simulink model "sus"  (Simulink 6.5)
settings: Solver=ode45  StartTime=0.0  StopTime=16  RelTol=1e-3
libraries: cdsFilt x266, cdsBitwise x92, cdsEpicsOut x84, cdsEpicsBinIn x56, cdsEpicsIn x20, cdsFiltCtrl x18, cdsMatrix x11, cdsSwitch x7, cdsWD x7, cdsFunctionCall x5, cdsRio1 x4, dac x3
(part 4 of 20)

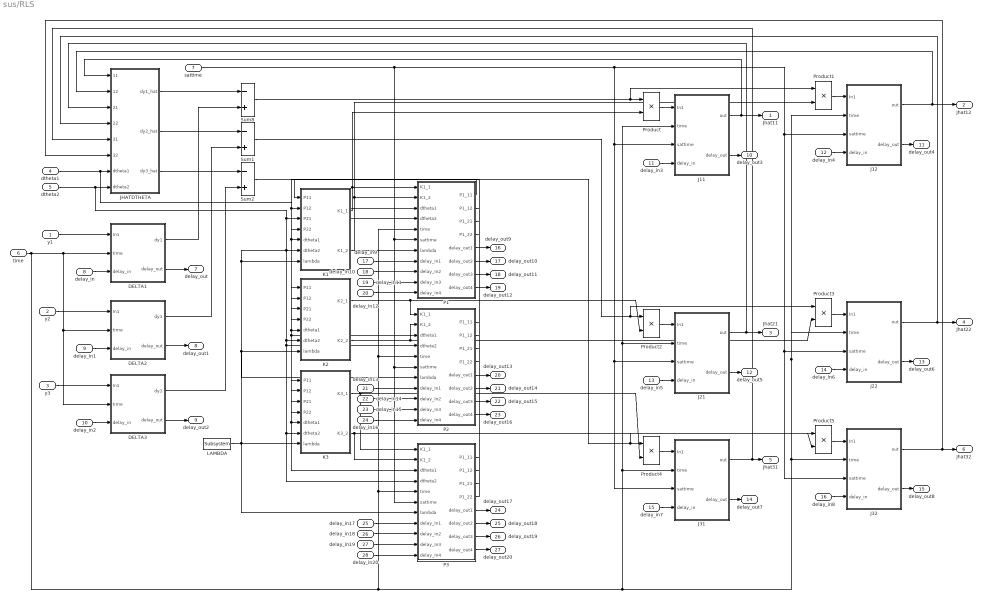
== system sus/RLS ==
  y1 : Inport
  y2 : Inport  Port=2
  y3 : Inport  Port=3
  dtheta1 : Inport  Port=4
  dtheta2 : Inport  Port=5
  time : Inport  Port=6
  sattime : Inport  Port=7
  delay_in : Inport  Port=8
  delay_in1 : Inport  Port=9
  delay_in2 : Inport  Port=10
  delay_in3 : Inport  Port=11
  delay_in4 : Inport  Port=12
  delay_in5 : Inport  Port=13
  delay_in6 : Inport  Port=14
  delay_in7 : Inport  Port=15
  delay_in8 : Inport  Port=16
  delay_in9 : Inport  Port=17
  delay_in10 : Inport  Port=18
  delay_in11 : Inport  Port=19
  delay_in12 : Inport  Port=20
  delay_in13 : Inport  Port=21
  delay_in14 : Inport  Port=22
  delay_in15 : Inport  Port=23
  delay_in16 : Inport  Port=24
  delay_in17 : Inport  Port=25
  delay_in18 : Inport  Port=26
  delay_in19 : Inport  Port=27
  delay_in20 : Inport  Port=28
  DELTA1 : Subsystem
  DELTA2 : Subsystem
  DELTA3 : Subsystem
  J11 : Subsystem
  J12 : Subsystem
  J21 : Subsystem
  J22 : Subsystem
  J31 : Subsystem
  J32 : Subsystem
  JHATDTHETA : Subsystem
  K1 : Subsystem
  K2 : Subsystem
  K3 : Subsystem
  LAMBDA : cdsEpicsIn/Subsystem  Tag=cdsEpicsIn  Description=|  SystemSampleTime=-1
      | Purpose:                                                                              
      | Create an EPICS input channel connection to the FE realtime controls.                 
      |                                                                                       
      | Operation:                                                                            
      | Outputs value from an EPICS ai record. Value is floating point with a precision of 3..
      |                                                                                       
      | Usage:                                                                                
      | Name the part with the desired EPICS channel name.
      settings: AttributesFormatString=%<Tag>
  P1 : Subsystem
  P2 : Subsystem
  P3 : Subsystem
  Product{,1..5} (6 alike) : Product  RndMeth=Zero
  Sum1 : Sum  Inputs=-+
  Sum2 : Sum  Inputs=-+
  Sum8 : Sum  Inputs=-+
  Jhat11 : Outport
  Jhat12 : Outport  Port=2
  Jhat21 : Outport  Port=3
  Jhat22 : Outport  Port=4
  Jhat31 : Outport  Port=5
  Jhat32 : Outport  Port=6
  delay_out : Outport  Port=7
  delay_out1 : Outport  Port=8
  delay_out2 : Outport  Port=9
  delay_out3 : Outport  Port=10
  delay_out4 : Outport  Port=11
  delay_out5 : Outport  Port=12
  delay_out6 : Outport  Port=13
  delay_out7 : Outport  Port=14
  delay_out8 : Outport  Port=15
  delay_out9 : Outport  Port=16
  delay_out10 : Outport  Port=17
  delay_out11 : Outport  Port=18
  delay_out12 : Outport  Port=19
  delay_out13 : Outport  Port=20
  delay_out14 : Outport  Port=21
  delay_out15 : Outport  Port=22
  delay_out16 : Outport  Port=23
  delay_out17 : Outport  Port=24
  delay_out18 : Outport  Port=25
  delay_out19 : Outport  Port=26
  delay_out20 : Outport  Port=27
  wires:
  time/1 -> DELTA1/2(time), DELTA2/2(time), DELTA3/2(time), J11/2(time), J21/2(time), J31/2(time), J12/2(time), J22/2(time), J32/2(time), P1/5(time), P2/5(time), P3/5(time)
  y1/1 -> DELTA1/1(In1)
  delay_in/1 -> DELTA1/3(delay_in)
  DELTA1/2(delay_out) -> delay_out/1
  y2/1 -> DELTA2/1(In1)
  delay_in1/1 -> DELTA2/3(delay_in)
  DELTA2/2(delay_out) -> delay_out1/1
  y3/1 -> DELTA3/1(In1)
  delay_in2/1 -> DELTA3/3(delay_in)
  DELTA3/2(delay_out) -> delay_out2/1
  dtheta1/1 -> JHATDTHETA/7(dtheta1), K1/5(dtheta1), K2/5(dtheta1), K3/5(dtheta1), P3/3(dtheta1), P2/3(dtheta1), P1/3(dtheta1)
  dtheta2/1 -> JHATDTHETA/8(dtheta2), K1/6(dtheta2), K2/6(dtheta2), K3/6(dtheta2), P3/4(dtheta2), P2/4(dtheta2), P1/4(dtheta2)
  JHATDTHETA/1(dy1_hat) -> Sum8/1
  DELTA1/1(dy1) -> Sum8/2
  JHATDTHETA/2(dy2_hat) -> Sum1/1
  DELTA2/1(dy1) -> Sum1/2
  JHATDTHETA/3(dy3_hat) -> Sum2/1
  DELTA3/1(dy1) -> Sum2/2
  delay_in3/1 -> J11/4(delay_in)
  J11/2(delay_out) -> delay_out3/1
  Product/1 -> J11/1(In1)
  delay_in4/1 -> J12/4(delay_in)
  J12/2(delay_out) -> delay_out4/1
  Product1/1 -> J12/1(In1)
  delay_in5/1 -> J21/4(delay_in)
  J21/2(delay_out) -> delay_out5/1
  Product2/1 -> J21/1(In1)
  delay_in6/1 -> J22/4(delay_in)
  J22/2(delay_out) -> delay_out6/1
  Product3/1 -> J22/1(In1)
  delay_in7/1 -> J31/4(delay_in)
  J31/2(delay_out) -> delay_out7/1
  Product4/1 -> J31/1(In1)
  delay_in8/1 -> J32/4(delay_in)
  J32/2(delay_out) -> delay_out8/1
  Product5/1 -> J32/1(In1)
  J11/1(out) -> Jhat11/1, JHATDTHETA/1(11)
  J12/1(out) -> Jhat12/1, JHATDTHETA/2(12)
  J21/1(out) -> Jhat21/1, JHATDTHETA/3(21)
  J22/1(out) -> Jhat22/1, JHATDTHETA/4(22)
  J31/1(out) -> Jhat31/1, JHATDTHETA/5(31)
  J32/1(out) -> Jhat32/1, JHATDTHETA/6(32)
  Sum8/1 -> Product/1, Product1/1
  Sum1/1 -> Product2/1, Product3/1
  Sum2/1 -> Product4/1, Product5/1
  sattime/1 -> J11/3(sattime), J21/3(sattime), J31/3(sattime), J22/3(sattime), J32/3(sattime), J12/3(sattime), P1/6(sattime), P2/6(sattime), P3/6(sattime)
  K1/1(K1_1) -> Product/2, P1/1(K1_1)
  K1/2(K1_2) -> Product1/2, P1/2(K1_2)
  K2/1(K2_1) -> Product2/2, P2/1(K1_1)
  K2/2(K2_2) -> Product3/2, P2/2(K1_2)
  K3/1(K3_1) -> Product4/2, P3/1(K1_1)
  K3/2(K3_2) -> Product5/2, P3/2(K1_2)
  LAMBDA/1 -> K3/7(lambda), K1/7(lambda), P1/7(lambda), K2/7(lambda), P2/7(lambda), P3/7(lambda)
  P1/1(P1_11) -> K1/1(P11)
  P1/2(P1_12) -> K1/2(P12)
  P1/3(P1_21) -> K1/3(P21)
  P1/4(P1_22) -> K1/4(P22)
  P2/1(P1_11) -> K2/1(P11)
  P2/2(P1_12) -> K2/2(P12)
  P2/3(P1_21) -> K2/3(P21)
  P2/4(P1_22) -> K2/4(P22)
  P3/1(P1_11) -> K3/1(P11)
  P3/2(P1_12) -> K3/2(P12)
  P3/3(P1_21) -> K3/3(P21)
  P3/4(P1_22) -> K3/4(P22)
  delay_in9/1 -> P1/8(delay_In1)
  P1/5(delay_out1) -> delay_out9/1
  delay_in10/1 -> P1/9(delay_In2)
  delay_in11/1 -> P1/10(delay_In3)
  delay_in12/1 -> P1/11(delay_In4)
  delay_in13/1 -> P2/8(delay_In1)
  delay_in14/1 -> P2/9(delay_In2)
  delay_in15/1 -> P2/10(delay_In3)
  delay_in16/1 -> P2/11(delay_In4)
  delay_in17/1 -> P3/8(delay_In1)
  delay_in18/1 -> P3/9(delay_In2)
  delay_in19/1 -> P3/10(delay_In3)
  delay_in20/1 -> P3/11(delay_In4)
  P1/6(delay_out2) -> delay_out10/1
  P1/7(delay_out3) -> delay_out11/1
  P1/8(delay_out4) -> delay_out12/1
  P2/5(delay_out1) -> delay_out13/1
  P2/6(delay_out2) -> delay_out14/1
  P2/7(delay_out3) -> delay_out15/1
  P2/8(delay_out4) -> delay_out16/1
  P3/5(delay_out1) -> delay_out17/1
  P3/6(delay_out2) -> delay_out18/1
  P3/7(delay_out3) -> delay_out19/1
  P3/8(delay_out4) -> delay_out20/1

== system sus/SATCLOCK ==
  In1 : Inport
  delay_in : Inport  Port=2
  Saturation : Saturate  UpperLimit=94.5+(1/16384)  LowerLimit=0
  Sum8 : Sum
  Out1 : Outport
  delay_out : Outport  Port=2
  wires:
  In1/1 -> Sum8/2
  Sum8/1 -> delay_out/1, Saturation/1
  delay_in/1 -> Sum8/1
  Saturation/1 -> Out1/1
